simulink model "SingleAgent_Manipulator"  (R2018b)
settings: Solver=VariableStepAuto  StartTime=0.0  StopTime=10  RelTol=1e-3
values from neighbouring files (symbols this model uses):
  Ts = 0.05; Simulation.Ts = Ts    [Parameters.m]
undefined symbols (not defined in the file or in its folder): p02, q01
settings Model: Creator=oscar  LastModifiedBy=oscar

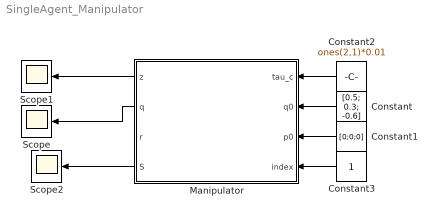
== system SingleAgent_Manipulator ==
  Constant : Constant  Value=[0.5; 0.3; -0.6]
  Constant1 : Constant  Value=[0;0;0]
  Constant2 : Constant  Value=ones(2,1)*0.01
  Constant3 : Constant
  Manipulator : Subsystem
  Scope : Scope
  Scope1 : Scope
  Scope2 : Scope
  wires:
  Constant/1 -> Manipulator/2(q0)
  Constant1/1 -> Manipulator/3(p0)
  Constant2/1 -> Manipulator/1(tau_c)
  Manipulator/2(q) -> Scope/1
  Manipulator/1(z) -> Scope1/1
  Constant3/1 -> Manipulator/4(index)
  Manipulator/4(S) -> Scope2/1

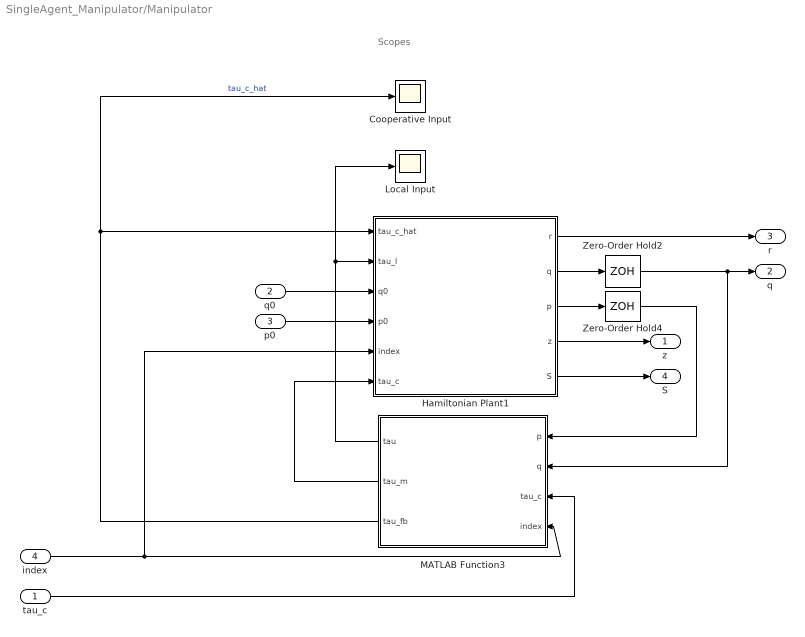
== system SingleAgent_Manipulator/Manipulator ==
  note: Scopes
  tau_c : Inport
  q0 : Inport  Port=2
  p0 : Inport  Port=3
  index : Inport  Port=4
  Cooperative Input : Scope
  Hamiltonian Plant1 : Subsystem
  Local Input : Scope
  MATLAB Function3 : MATLAB Function  TreatAsAtomicUnit=on
  Zero-Order Hold2 : ZeroOrderHold  SampleTime=Ts
  Zero-Order Hold4 : ZeroOrderHold  SampleTime=Ts
  z : Outport
  q : Outport  Port=2
  r : Outport  Port=3
  S : Outport  Port=4
  wires:
  tau_c/1 -> MATLAB Function3/3(tau_c)
  Hamiltonian Plant1/5(S) -> S/1
  Hamiltonian Plant1/2(q) -> Zero-Order Hold2/1
  index/1 -> Hamiltonian Plant1/5(index), MATLAB Function3/4(index)
  Hamiltonian Plant1/1(r) -> r/1
  MATLAB Function3/1(tau) -> Hamiltonian Plant1/2(tau_l), Local Input/1
  Hamiltonian Plant1/4(z) -> z/1
  p0/1 -> Hamiltonian Plant1/4(p0)
  MATLAB Function3/3(tau_fb) -> Hamiltonian Plant1/1(tau_c_hat), Cooperative Input/1  "tau_c_hat"
  MATLAB Function3/2(tau_m) -> Hamiltonian Plant1/6(tau_c)
  Hamiltonian Plant1/3(p) -> Zero-Order Hold4/1
  q0/1 -> Hamiltonian Plant1/3(q0)
  Zero-Order Hold2/1 -> MATLAB Function3/2(q), q/1
  Zero-Order Hold4/1 -> MATLAB Function3/1(p)

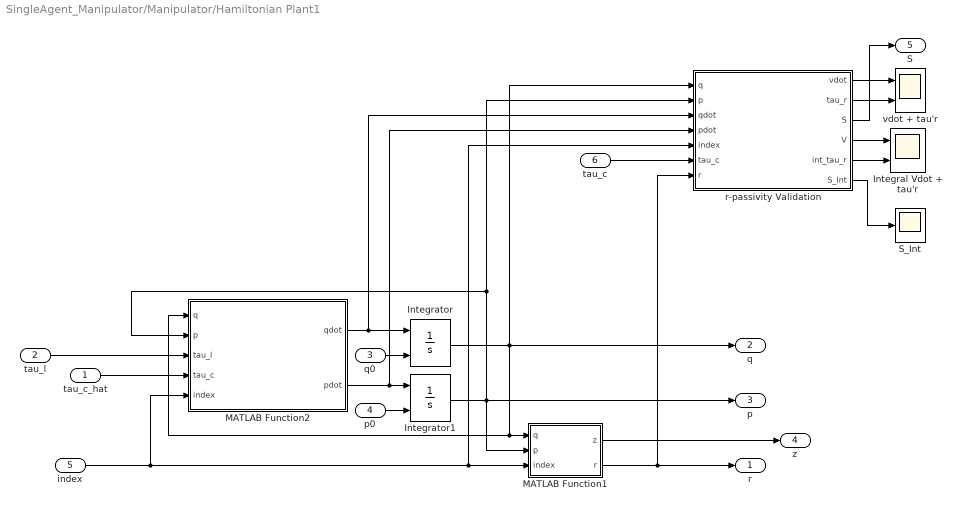
== system SingleAgent_Manipulator/Manipulator/Hamiltonian Plant1 ==
  tau_c_hat : Inport
  tau_l : Inport  Port=2
  q0 : Inport  Port=3
  p0 : Inport  Port=4
  index : Inport  Port=5
  tau_c : Inport  Port=6
  Integral Vdot + tau'r : Scope  NumInputPorts=2
  Integrator : Integrator  InitialConditionSource=external  InitialCondition=q01
  Integrator1 : Integrator  InitialConditionSource=external  InitialCondition=p02
  MATLAB Function1 : MATLAB Function  TreatAsAtomicUnit=on
  MATLAB Function2 : MATLAB Function  TreatAsAtomicUnit=on
  S_Int : Scope
  r-passivity Validation : Subsystem
  vdot + tau'r : Scope  NumInputPorts=2
  r : Outport
  q : Outport  Port=2
  p : Outport  Port=3
  z : Outport  Port=4
  S : Outport  Port=5
  wires:
  tau_l/1 -> MATLAB Function2/3(tau_l)
  MATLAB Function2/2(pdot) -> r-passivity Validation/4(pdot), Integrator1/1
  Integrator1/1 -> r-passivity Validation/2(p), MATLAB Function2/2(p), p/1, MATLAB Function1/2(p)
  Integrator/1 -> r-passivity Validation/1(q), q/1, MATLAB Function2/1(q), MATLAB Function1/1(q)
  MATLAB Function2/1(qdot) -> r-passivity Validation/3(qdot), Integrator/1
  p0/1 -> Integrator1/2
  q0/1 -> Integrator/2
  MATLAB Function1/1(z) -> z/1
  MATLAB Function1/2(r) -> r-passivity Validation/7(r), r/1
  index/1 -> r-passivity Validation/5(index), MATLAB Function1/3(index), MATLAB Function2/5(index)
  r-passivity Validation/1(vdot) -> vdot + tau'r/1
  r-passivity Validation/2(tau_r) -> vdot + tau'r/2
  r-passivity Validation/5(int_tau_r) -> Integral Vdot + tau'r/2
  r-passivity Validation/4(V) -> Integral Vdot + tau'r/1
  r-passivity Validation/3(S) -> S/1
  tau_c/1 -> r-passivity Validation/6(tau_c)
  tau_c_hat/1 -> MATLAB Function2/4(tau_c)
  r-passivity Validation/6(S_Int) -> S_Int/1

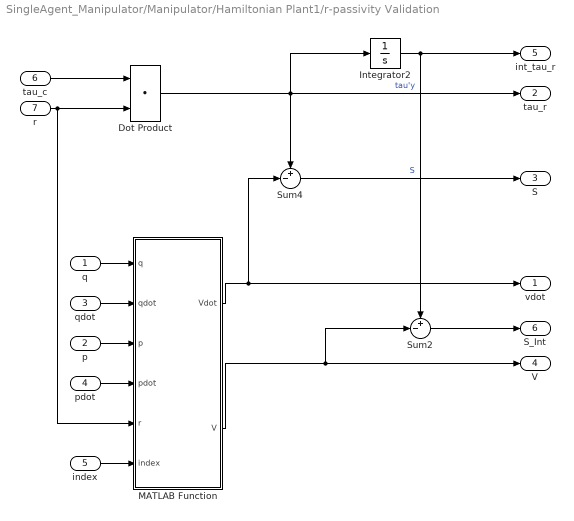
== system SingleAgent_Manipulator/Manipulator/Hamiltonian Plant1/r-passivity Validation ==
  q : Inport
  p : Inport  Port=2
  qdot : Inport  Port=3
  pdot : Inport  Port=4
  index : Inport  Port=5
  tau_c : Inport  Port=6
  r : Inport  Port=7
  Dot Product : DotProduct  InputSameDT=on  OutDataTypeStr=Inherit: Inherit via internal rule
  Integrator2 : Integrator
  MATLAB Function : MATLAB Function  TreatAsAtomicUnit=on
  Sum2 : Sum  Inputs=+-|
  Sum4 : Sum  Inputs=+-|
  vdot : Outport
  tau_r : Outport  Port=2
  S : Outport  Port=3
  V : Outport  Port=4
  int_tau_r : Outport  Port=5
  S_Int : Outport  Port=6
  wires:
  Sum4/1 -> S/1  "S"
  pdot/1 -> MATLAB Function/4(pdot)
  p/1 -> MATLAB Function/3(p)
  qdot/1 -> MATLAB Function/2(qdot)
  index/1 -> MATLAB Function/6(index)
  q/1 -> MATLAB Function/1(q)
  tau_c/1 -> Dot Product/1
  r/1 -> Dot Product/2, MATLAB Function/5(r)
  Dot Product/1 -> Integrator2/1, tau_r/1, Sum4/1  "tau'y"
  MATLAB Function/1(Vdot) -> Sum4/2, vdot/1
  MATLAB Function/2(V) -> Sum2/2, V/1
  Integrator2/1 -> int_tau_r/1, Sum2/1
  Sum2/1 -> S_Int/1

== matlab function SingleAgent_Manipulator/Manipulator/Hamiltonian Plant1/MATLAB Function1 ==
  data: q input; z output; p input; r output; index input
function [z, r] = toz(q, p, index)

    coder.extrinsic('Manipulator_z');
    z = zeros(2, 1);
    r = zeros(2, 1);
    [z, r] = Manipulator_z(q, p, index);

== matlab function SingleAgent_Manipulator/Manipulator/Hamiltonian Plant1/MATLAB Function2 ==
  data: q input; qdot output; p input; tau_l input; pdot output; tau_c input; index input
function [qdot, pdot] = fcn(q, p, tau_l, tau_c, index)

    coder.extrinsic('Manipulator_Dynamics');
    qdot = zeros(3, 1);
    pdot = zeros(3, 1);
    [qdot, pdot] = Manipulator_Dynamics(q, p, tau_l, tau_c, index);

== matlab function SingleAgent_Manipulator/Manipulator/Hamiltonian Plant1/r-passivity Validation/MATLAB Function ==
  data: Vdot output; q input; qdot input; p input; pdot input; r input; index input; V output
function [Vdot, V] = fcn(q, qdot, p, pdot, r, index)

    coder.extrinsic('Manipulator_R');
    V = 0; Vdot = 0;
    [V, Vdot] = Manipulator_R(q, qdot,p, pdot, r, index);
end

== matlab function SingleAgent_Manipulator/Manipulator/MATLAB Function3 ==
  data: p input; q input; tau_c input; tau output; tau_m output; tau_fb output; index input
function [tau, tau_m, tau_fb] = LocalControl(p, q, tau_c, index)
    

coder.extrinsic('Manipulator_Control');
tau = zeros(3, 1);
tau_fb = zeros(2, 1);
tau_m = zeros(2, 1);
[tau, tau_m, tau_fb] = Manipulator_Control(q, p, tau_c, index);
